simulink model "final"  (R2014a)
settings: Solver=FixedStepDiscrete  StartTime=0.0  StopTime=50000  FixedStep=1  RelTol=1e-3
libraries: hdlsllib x15, simulink x5
settings Model: Creator=you.r  LastModifiedBy=sheehan.pat
settings OptimizationCC: BlockReduction=off  ConditionallyExecuteInputs=off  InlineParams=on
settings DebuggingCC: AlgebraicLoopMsg=error
settings HardwareCC: ProdHWDeviceType=ASIC/FPGA->ASIC/FPGA  ProdEqTarget=off

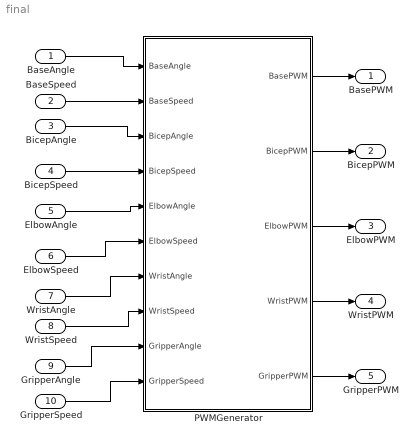
== system final ==
  BaseAngle : Inport
  BaseSpeed : Inport  Port=2
  BicepAngle : Inport  Port=3
  BicepSpeed : Inport  Port=4
  ElbowAngle : Inport  Port=5
  ElbowSpeed : Inport  Port=6
  WristAngle : Inport  Port=7
  WristSpeed : Inport  Port=8
  GripperAngle : Inport  Port=9
  GripperSpeed : Inport  Port=10
  PWMGenerator : Subsystem  TreatAsAtomicUnit=on  SystemSampleTime=1
  BasePWM : Outport  OutDataTypeStr=boolean  SampleTime=1
  BicepPWM : Outport  Port=2  OutDataTypeStr=boolean  SampleTime=1
  ElbowPWM : Outport  Port=3  OutDataTypeStr=boolean  SampleTime=1
  WristPWM : Outport  Port=4  OutDataTypeStr=boolean  SampleTime=1
  GripperPWM : Outport  Port=5  OutDataTypeStr=boolean  SampleTime=1
  wires:
  PWMGenerator/1(BasePWM) -> BasePWM/1
  PWMGenerator/2(BicepPWM) -> BicepPWM/1
  PWMGenerator/3(ElbowPWM) -> ElbowPWM/1
  PWMGenerator/4(WristPWM) -> WristPWM/1
  PWMGenerator/5(GripperPWM) -> GripperPWM/1
  ElbowAngle/1 -> PWMGenerator/5(ElbowAngle)
  ElbowSpeed/1 -> PWMGenerator/6(ElbowSpeed)
  BicepSpeed/1 -> PWMGenerator/4(BicepSpeed)
  BicepAngle/1 -> PWMGenerator/3(BicepAngle)
  WristAngle/1 -> PWMGenerator/7(WristAngle)
  WristSpeed/1 -> PWMGenerator/8(WristSpeed)
  BaseSpeed/1 -> PWMGenerator/2(BaseSpeed)
  BaseAngle/1 -> PWMGenerator/1(BaseAngle)
  GripperAngle/1 -> PWMGenerator/9(GripperAngle)
  GripperSpeed/1 -> PWMGenerator/10(GripperSpeed)

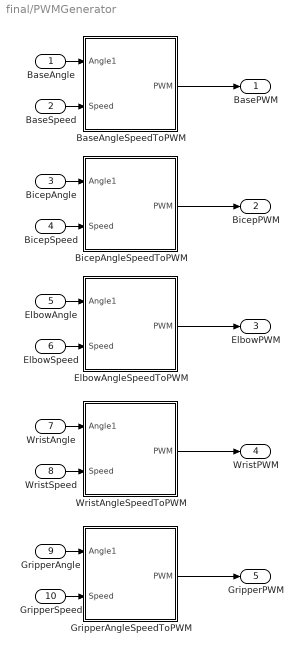
== system final/PWMGenerator ==
  BaseAngle : Inport
  BaseSpeed : Inport  Port=2
  BicepAngle : Inport  Port=3
  BicepSpeed : Inport  Port=4
  ElbowAngle : Inport  Port=5
  ElbowSpeed : Inport  Port=6
  WristAngle : Inport  Port=7
  WristSpeed : Inport  Port=8
  GripperAngle : Inport  Port=9
  GripperSpeed : Inport  Port=10
  BaseAngleSpeedToPWM : Subsystem  TreatAsAtomicUnit=on  SystemSampleTime=1
  BicepAngleSpeedToPWM : Subsystem  TreatAsAtomicUnit=on  SystemSampleTime=1
  ElbowAngleSpeedToPWM : Subsystem  TreatAsAtomicUnit=on  SystemSampleTime=1
  GripperAngleSpeedToPWM : Subsystem  TreatAsAtomicUnit=on  SystemSampleTime=1
  WristAngleSpeedToPWM : Subsystem  TreatAsAtomicUnit=on  SystemSampleTime=1
  BasePWM : Outport  OutDataTypeStr=boolean  SampleTime=1
  BicepPWM : Outport  Port=2  OutDataTypeStr=boolean  SampleTime=1
  ElbowPWM : Outport  Port=3  OutDataTypeStr=boolean  SampleTime=1
  WristPWM : Outport  Port=4  OutDataTypeStr=boolean  SampleTime=1
  GripperPWM : Outport  Port=5  OutDataTypeStr=boolean  SampleTime=1
  wires:
  BaseAngleSpeedToPWM/1(PWM) -> BasePWM/1
  GripperAngleSpeedToPWM/1(PWM) -> GripperPWM/1
  ElbowSpeed/1 -> ElbowAngleSpeedToPWM/2(Speed)
  BaseSpeed/1 -> BaseAngleSpeedToPWM/2(Speed)
  GripperAngle/1 -> GripperAngleSpeedToPWM/1(Angle1)
  WristSpeed/1 -> WristAngleSpeedToPWM/2(Speed)
  BicepSpeed/1 -> BicepAngleSpeedToPWM/2(Speed)
  ElbowAngle/1 -> ElbowAngleSpeedToPWM/1(Angle1)
  GripperSpeed/1 -> GripperAngleSpeedToPWM/2(Speed)
  BaseAngle/1 -> BaseAngleSpeedToPWM/1(Angle1)
  WristAngle/1 -> WristAngleSpeedToPWM/1(Angle1)
  BicepAngle/1 -> BicepAngleSpeedToPWM/1(Angle1)
  BicepAngleSpeedToPWM/1(PWM) -> BicepPWM/1
  ElbowAngleSpeedToPWM/1(PWM) -> ElbowPWM/1
  WristAngleSpeedToPWM/1(PWM) -> WristPWM/1

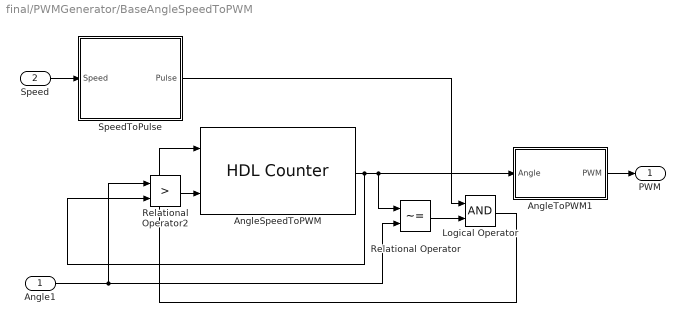
== system final/PWMGenerator/BaseAngleSpeedToPWM ==
  Angle1 : Inport  OutDataTypeStr=uint8
  Speed : Inport  Port=2  OutDataTypeStr=uint8
  AngleSpeedToPWM : hdlsllib/HDL Operations/HDL Counter  CountType=Count limited  CountInit=90  CountStep=1  CountMax=180  CountFromType=Initial value  CountFrom=90  CountResetPort=off  CountLoadPort=off  CountEnbPort=on  CountDirPort=on  CountDataType=Unsigned  CountWordLen=8  CountFracLen=0  CountSampTime=1
  AngleToPWM1 : Subsystem
  Logical Operator : Logic  AllPortsSameDT=off  OutDataTypeStr=boolean
  Relational Operator : RelationalOperator  Operator=~=  OutDataTypeStr=boolean
  Relational Operator2 : RelationalOperator  Operator=>  OutDataTypeStr=boolean
  SpeedToPulse : Subsystem
  PWM : Outport  OutDataTypeStr=boolean  SampleTime=1
  wires:
  Relational Operator/1 -> Logical Operator/2
  AngleSpeedToPWM/1 -> Relational Operator2/2, AngleToPWM1/1(Angle), Relational Operator/1
  Angle1/1 -> Relational Operator2/1, Relational Operator/2
  Relational Operator2/1 -> AngleSpeedToPWM/2
  Logical Operator/1 -> AngleSpeedToPWM/1
  SpeedToPulse/1(Pulse) -> Logical Operator/1
  Speed/1 -> SpeedToPulse/1(Speed)
  AngleToPWM1/1(PWM) -> PWM/1

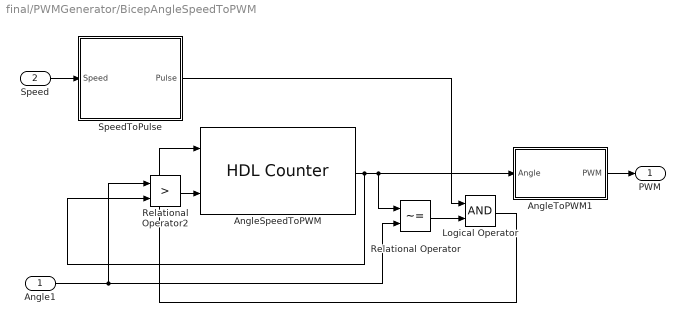
== system final/PWMGenerator/BicepAngleSpeedToPWM ==
  Angle1 : Inport  OutDataTypeStr=uint8
  Speed : Inport  Port=2  OutDataTypeStr=uint8
  AngleSpeedToPWM : hdlsllib/HDL Operations/HDL Counter  CountType=Count limited  CountInit=90  CountStep=1  CountMax=180  CountFromType=Initial value  CountFrom=90  CountResetPort=off  CountLoadPort=off  CountEnbPort=on  CountDirPort=on  CountDataType=Unsigned  CountWordLen=8  CountFracLen=0  CountSampTime=1
  AngleToPWM1 : Subsystem
  Logical Operator : Logic  AllPortsSameDT=off  OutDataTypeStr=boolean
  Relational Operator : RelationalOperator  Operator=~=  OutDataTypeStr=boolean
  Relational Operator2 : RelationalOperator  Operator=>  OutDataTypeStr=boolean
  SpeedToPulse : Subsystem
  PWM : Outport  OutDataTypeStr=boolean  SampleTime=1
  wires:
  Relational Operator/1 -> Logical Operator/2
  AngleSpeedToPWM/1 -> Relational Operator2/2, AngleToPWM1/1(Angle), Relational Operator/1
  Angle1/1 -> Relational Operator2/1, Relational Operator/2
  Relational Operator2/1 -> AngleSpeedToPWM/2
  Logical Operator/1 -> AngleSpeedToPWM/1
  SpeedToPulse/1(Pulse) -> Logical Operator/1
  Speed/1 -> SpeedToPulse/1(Speed)
  AngleToPWM1/1(PWM) -> PWM/1

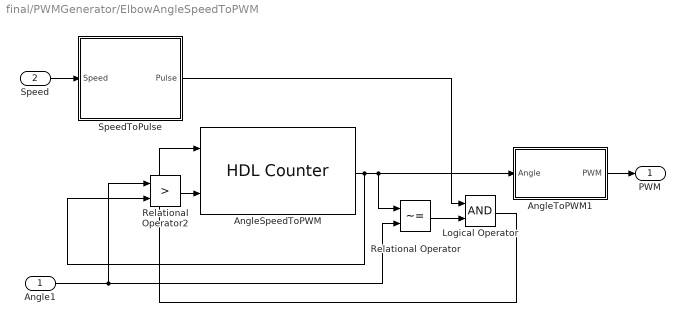
== system final/PWMGenerator/ElbowAngleSpeedToPWM ==
  Angle1 : Inport  OutDataTypeStr=uint8
  Speed : Inport  Port=2  OutDataTypeStr=uint8
  AngleSpeedToPWM : hdlsllib/HDL Operations/HDL Counter  CountType=Count limited  CountInit=90  CountStep=1  CountMax=180  CountFromType=Initial value  CountFrom=90  CountResetPort=off  CountLoadPort=off  CountEnbPort=on  CountDirPort=on  CountDataType=Unsigned  CountWordLen=8  CountFracLen=0  CountSampTime=1
  AngleToPWM1 : Subsystem
  Logical Operator : Logic  AllPortsSameDT=off  OutDataTypeStr=boolean
  Relational Operator : RelationalOperator  Operator=~=  OutDataTypeStr=boolean
  Relational Operator2 : RelationalOperator  Operator=>  OutDataTypeStr=boolean
  SpeedToPulse : Subsystem
  PWM : Outport  OutDataTypeStr=boolean  SampleTime=1
  wires:
  Relational Operator/1 -> Logical Operator/2
  AngleSpeedToPWM/1 -> Relational Operator2/2, AngleToPWM1/1(Angle), Relational Operator/1
  Angle1/1 -> Relational Operator2/1, Relational Operator/2
  Relational Operator2/1 -> AngleSpeedToPWM/2
  Logical Operator/1 -> AngleSpeedToPWM/1
  SpeedToPulse/1(Pulse) -> Logical Operator/1
  Speed/1 -> SpeedToPulse/1(Speed)
  AngleToPWM1/1(PWM) -> PWM/1

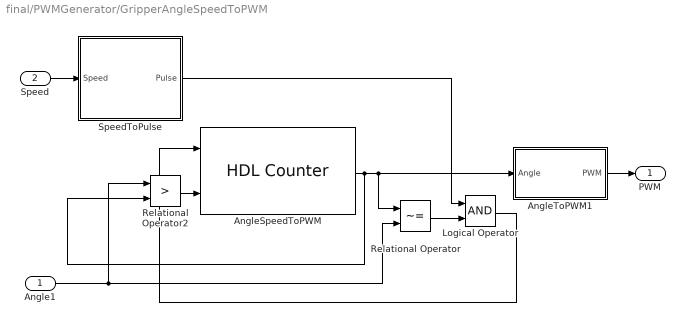
== system final/PWMGenerator/GripperAngleSpeedToPWM ==
  Angle1 : Inport  OutDataTypeStr=uint8
  Speed : Inport  Port=2  OutDataTypeStr=uint8
  AngleSpeedToPWM : hdlsllib/HDL Operations/HDL Counter  CountType=Count limited  CountInit=90  CountStep=1  CountMax=180  CountFromType=Initial value  CountFrom=90  CountResetPort=off  CountLoadPort=off  CountEnbPort=on  CountDirPort=on  CountDataType=Unsigned  CountWordLen=8  CountFracLen=0  CountSampTime=1
  AngleToPWM1 : Subsystem
  Logical Operator : Logic  AllPortsSameDT=off  OutDataTypeStr=boolean
  Relational Operator : RelationalOperator  Operator=~=  OutDataTypeStr=boolean
  Relational Operator2 : RelationalOperator  Operator=>  OutDataTypeStr=boolean
  SpeedToPulse : Subsystem
  PWM : Outport  OutDataTypeStr=boolean  SampleTime=1
  wires:
  Relational Operator/1 -> Logical Operator/2
  AngleSpeedToPWM/1 -> Relational Operator2/2, AngleToPWM1/1(Angle), Relational Operator/1
  Angle1/1 -> Relational Operator2/1, Relational Operator/2
  Relational Operator2/1 -> AngleSpeedToPWM/2
  Logical Operator/1 -> AngleSpeedToPWM/1
  SpeedToPulse/1(Pulse) -> Logical Operator/1
  Speed/1 -> SpeedToPulse/1(Speed)
  AngleToPWM1/1(PWM) -> PWM/1

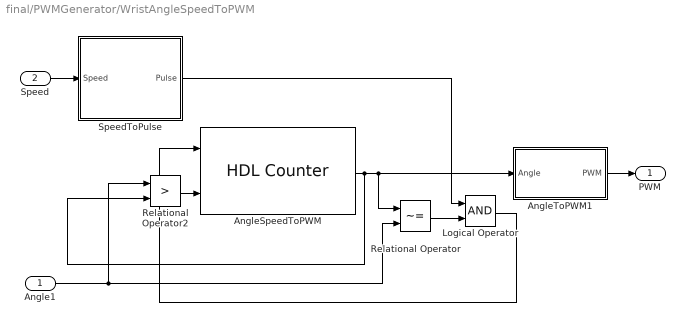
== system final/PWMGenerator/WristAngleSpeedToPWM ==
  Angle1 : Inport  OutDataTypeStr=uint8
  Speed : Inport  Port=2  OutDataTypeStr=uint8
  AngleSpeedToPWM : hdlsllib/HDL Operations/HDL Counter  CountType=Count limited  CountInit=90  CountStep=1  CountMax=180  CountFromType=Initial value  CountFrom=90  CountResetPort=off  CountLoadPort=off  CountEnbPort=on  CountDirPort=on  CountDataType=Unsigned  CountWordLen=8  CountFracLen=0  CountSampTime=1
  AngleToPWM1 : Subsystem
  Logical Operator : Logic  AllPortsSameDT=off  OutDataTypeStr=boolean
  Relational Operator : RelationalOperator  Operator=~=  OutDataTypeStr=boolean
  Relational Operator2 : RelationalOperator  Operator=>  OutDataTypeStr=boolean
  SpeedToPulse : Subsystem
  PWM : Outport  OutDataTypeStr=boolean  SampleTime=1
  wires:
  Relational Operator/1 -> Logical Operator/2
  AngleSpeedToPWM/1 -> Relational Operator2/2, AngleToPWM1/1(Angle), Relational Operator/1
  Angle1/1 -> Relational Operator2/1, Relational Operator/2
  Relational Operator2/1 -> AngleSpeedToPWM/2
  Logical Operator/1 -> AngleSpeedToPWM/1
  SpeedToPulse/1(Pulse) -> Logical Operator/1
  Speed/1 -> SpeedToPulse/1(Speed)
  AngleToPWM1/1(PWM) -> PWM/1

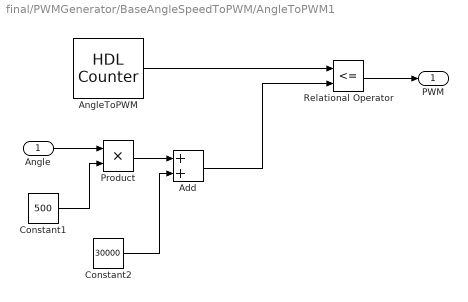
== system final/PWMGenerator/BaseAngleSpeedToPWM/AngleToPWM1 ==
  Angle : Inport  OutDataTypeStr=uint8
  Add : Sum
  AngleToPWM : hdlsllib/HDL Operations/HDL Counter  CountType=Count limited  CountInit=0  CountStep=1  CountMax=1000000  CountFromType=Initial value  CountFrom=0  CountResetPort=off  CountLoadPort=off  CountEnbPort=off  CountDirPort=off  CountDataType=Unsigned  CountWordLen=32  CountFracLen=0  CountSampTime=1
  Constant1 : Constant  Value=500  OutDataTypeStr=uint32  SampleTime=-1
  Constant2 : Constant  Value=30000  OutDataTypeStr=uint32  SampleTime=-1
  Product : Product
  Relational Operator : RelationalOperator  Operator=<=  OutDataTypeStr=boolean
  PWM : Outport
  wires:
  AngleToPWM/1 -> Relational Operator/1
  Angle/1 -> Product/1
  Relational Operator/1 -> PWM/1
  Constant1/1 -> Product/2
  Add/1 -> Relational Operator/2
  Constant2/1 -> Add/2
  Product/1 -> Add/1

== system final/PWMGenerator/BaseAngleSpeedToPWM/SpeedToPulse ==
  Speed : Inport
  Compare To Constant : simulink/Logic and Bit Operations/Compare To Constant  relop===  const=0  OutDataTypeStr=boolean
  Constant : Constant  Value=50000000  OutDataTypeStr=uint32  SampleTime=1
  Divide : Product  Inputs=*/  SaturateOnIntegerOverflow=on  RndMeth=Zero
  HDL Counter : hdlsllib/HDL Operations/HDL Counter  CountType=Free running  CountInit=0  CountStep=1  CountMax=100  CountFromType=Initial value  CountFrom=0  CountResetPort=on  CountLoadPort=off  CountEnbPort=off  CountDirPort=off  CountDataType=Unsigned  CountWordLen=32  CountFracLen=0  CountSampTime=1
  Relational Operator : RelationalOperator  Operator=>  OutDataTypeStr=boolean  SampleTime=1
  Pulse : Outport  OutDataTypeStr=boolean  SampleTime=1
  wires:
  Relational Operator/1 -> HDL Counter/1
  Compare To Constant/1 -> Pulse/1
  Constant/1 -> Divide/1
  Divide/1 -> Relational Operator/2
  HDL Counter/1 -> Relational Operator/1, Compare To Constant/1
  Speed/1 -> Divide/2

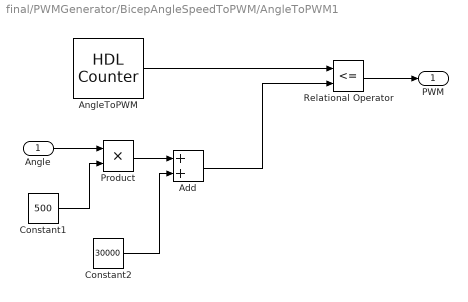
== system final/PWMGenerator/BicepAngleSpeedToPWM/AngleToPWM1 ==
  Angle : Inport  OutDataTypeStr=uint8
  Add : Sum
  AngleToPWM : hdlsllib/HDL Operations/HDL Counter  CountType=Count limited  CountInit=0  CountStep=1  CountMax=1000000  CountFromType=Initial value  CountFrom=0  CountResetPort=off  CountLoadPort=off  CountEnbPort=off  CountDirPort=off  CountDataType=Unsigned  CountWordLen=32  CountFracLen=0  CountSampTime=1
  Constant1 : Constant  Value=500  OutDataTypeStr=uint32  SampleTime=-1
  Constant2 : Constant  Value=30000  OutDataTypeStr=uint32  SampleTime=-1
  Product : Product
  Relational Operator : RelationalOperator  Operator=<=  OutDataTypeStr=boolean
  PWM : Outport
  wires:
  AngleToPWM/1 -> Relational Operator/1
  Angle/1 -> Product/1
  Relational Operator/1 -> PWM/1
  Constant1/1 -> Product/2
  Add/1 -> Relational Operator/2
  Constant2/1 -> Add/2
  Product/1 -> Add/1

== system final/PWMGenerator/BicepAngleSpeedToPWM/SpeedToPulse ==
  Speed : Inport
  Compare To Constant : simulink/Logic and Bit Operations/Compare To Constant  relop===  const=0  OutDataTypeStr=boolean
  Constant : Constant  Value=50000000  OutDataTypeStr=uint32  SampleTime=1
  Divide : Product  Inputs=*/  SaturateOnIntegerOverflow=on  RndMeth=Zero
  HDL Counter : hdlsllib/HDL Operations/HDL Counter  CountType=Free running  CountInit=0  CountStep=1  CountMax=100  CountFromType=Initial value  CountFrom=0  CountResetPort=on  CountLoadPort=off  CountEnbPort=off  CountDirPort=off  CountDataType=Unsigned  CountWordLen=32  CountFracLen=0  CountSampTime=1
  Relational Operator : RelationalOperator  Operator=>  OutDataTypeStr=boolean  SampleTime=1
  Pulse : Outport  OutDataTypeStr=boolean  SampleTime=1
  wires:
  Relational Operator/1 -> HDL Counter/1
  Compare To Constant/1 -> Pulse/1
  Constant/1 -> Divide/1
  Divide/1 -> Relational Operator/2
  HDL Counter/1 -> Relational Operator/1, Compare To Constant/1
  Speed/1 -> Divide/2

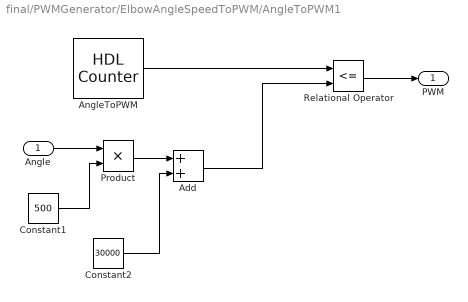
== system final/PWMGenerator/ElbowAngleSpeedToPWM/AngleToPWM1 ==
  Angle : Inport  OutDataTypeStr=uint8
  Add : Sum
  AngleToPWM : hdlsllib/HDL Operations/HDL Counter  CountType=Count limited  CountInit=0  CountStep=1  CountMax=1000000  CountFromType=Initial value  CountFrom=0  CountResetPort=off  CountLoadPort=off  CountEnbPort=off  CountDirPort=off  CountDataType=Unsigned  CountWordLen=32  CountFracLen=0  CountSampTime=1
  Constant1 : Constant  Value=500  OutDataTypeStr=uint32  SampleTime=-1
  Constant2 : Constant  Value=30000  OutDataTypeStr=uint32  SampleTime=-1
  Product : Product
  Relational Operator : RelationalOperator  Operator=<=  OutDataTypeStr=boolean
  PWM : Outport
  wires:
  AngleToPWM/1 -> Relational Operator/1
  Angle/1 -> Product/1
  Relational Operator/1 -> PWM/1
  Constant1/1 -> Product/2
  Add/1 -> Relational Operator/2
  Constant2/1 -> Add/2
  Product/1 -> Add/1

== system final/PWMGenerator/ElbowAngleSpeedToPWM/SpeedToPulse ==
  Speed : Inport
  Compare To Constant : simulink/Logic and Bit Operations/Compare To Constant  relop===  const=0  OutDataTypeStr=boolean
  Constant : Constant  Value=50000000  OutDataTypeStr=uint32  SampleTime=1
  Divide : Product  Inputs=*/  SaturateOnIntegerOverflow=on  RndMeth=Zero
  HDL Counter : hdlsllib/HDL Operations/HDL Counter  CountType=Free running  CountInit=0  CountStep=1  CountMax=100  CountFromType=Initial value  CountFrom=0  CountResetPort=on  CountLoadPort=off  CountEnbPort=off  CountDirPort=off  CountDataType=Unsigned  CountWordLen=32  CountFracLen=0  CountSampTime=1
  Relational Operator : RelationalOperator  Operator=>  OutDataTypeStr=boolean  SampleTime=1
  Pulse : Outport  OutDataTypeStr=boolean  SampleTime=1
  wires:
  Relational Operator/1 -> HDL Counter/1
  Compare To Constant/1 -> Pulse/1
  Constant/1 -> Divide/1
  Divide/1 -> Relational Operator/2
  HDL Counter/1 -> Relational Operator/1, Compare To Constant/1
  Speed/1 -> Divide/2

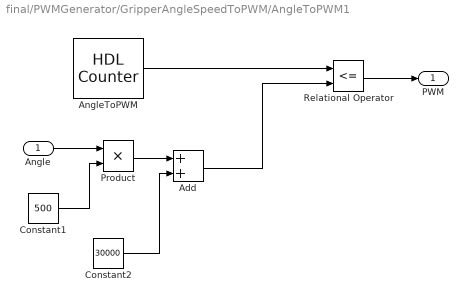
== system final/PWMGenerator/GripperAngleSpeedToPWM/AngleToPWM1 ==
  Angle : Inport  OutDataTypeStr=uint8
  Add : Sum
  AngleToPWM : hdlsllib/HDL Operations/HDL Counter  CountType=Count limited  CountInit=0  CountStep=1  CountMax=1000000  CountFromType=Initial value  CountFrom=0  CountResetPort=off  CountLoadPort=off  CountEnbPort=off  CountDirPort=off  CountDataType=Unsigned  CountWordLen=32  CountFracLen=0  CountSampTime=1
  Constant1 : Constant  Value=500  OutDataTypeStr=uint32  SampleTime=-1
  Constant2 : Constant  Value=30000  OutDataTypeStr=uint32  SampleTime=-1
  Product : Product
  Relational Operator : RelationalOperator  Operator=<=  OutDataTypeStr=boolean
  PWM : Outport
  wires:
  AngleToPWM/1 -> Relational Operator/1
  Angle/1 -> Product/1
  Relational Operator/1 -> PWM/1
  Constant1/1 -> Product/2
  Add/1 -> Relational Operator/2
  Constant2/1 -> Add/2
  Product/1 -> Add/1

== system final/PWMGenerator/GripperAngleSpeedToPWM/SpeedToPulse ==
  Speed : Inport
  Compare To Constant : simulink/Logic and Bit Operations/Compare To Constant  relop===  const=0  OutDataTypeStr=boolean
  Constant : Constant  Value=50000000  OutDataTypeStr=uint32  SampleTime=1
  Divide : Product  Inputs=*/  SaturateOnIntegerOverflow=on  RndMeth=Zero
  HDL Counter : hdlsllib/HDL Operations/HDL Counter  CountType=Free running  CountInit=0  CountStep=1  CountMax=100  CountFromType=Initial value  CountFrom=0  CountResetPort=on  CountLoadPort=off  CountEnbPort=off  CountDirPort=off  CountDataType=Unsigned  CountWordLen=32  CountFracLen=0  CountSampTime=1
  Relational Operator : RelationalOperator  Operator=>  OutDataTypeStr=boolean  SampleTime=1
  Pulse : Outport  OutDataTypeStr=boolean  SampleTime=1
  wires:
  Relational Operator/1 -> HDL Counter/1
  Compare To Constant/1 -> Pulse/1
  Constant/1 -> Divide/1
  Divide/1 -> Relational Operator/2
  HDL Counter/1 -> Relational Operator/1, Compare To Constant/1
  Speed/1 -> Divide/2

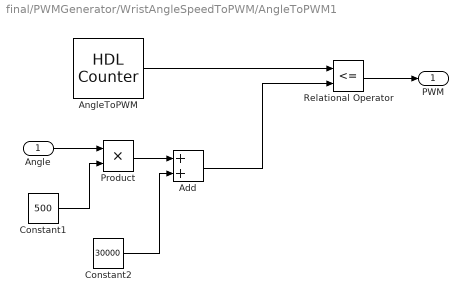
== system final/PWMGenerator/WristAngleSpeedToPWM/AngleToPWM1 ==
  Angle : Inport  OutDataTypeStr=uint8
  Add : Sum
  AngleToPWM : hdlsllib/HDL Operations/HDL Counter  CountType=Count limited  CountInit=0  CountStep=1  CountMax=1000000  CountFromType=Initial value  CountFrom=0  CountResetPort=off  CountLoadPort=off  CountEnbPort=off  CountDirPort=off  CountDataType=Unsigned  CountWordLen=32  CountFracLen=0  CountSampTime=1
  Constant1 : Constant  Value=500  OutDataTypeStr=uint32  SampleTime=-1
  Constant2 : Constant  Value=30000  OutDataTypeStr=uint32  SampleTime=-1
  Product : Product
  Relational Operator : RelationalOperator  Operator=<=  OutDataTypeStr=boolean
  PWM : Outport
  wires:
  AngleToPWM/1 -> Relational Operator/1
  Angle/1 -> Product/1
  Relational Operator/1 -> PWM/1
  Constant1/1 -> Product/2
  Add/1 -> Relational Operator/2
  Constant2/1 -> Add/2
  Product/1 -> Add/1

== system final/PWMGenerator/WristAngleSpeedToPWM/SpeedToPulse ==
  Speed : Inport
  Compare To Constant : simulink/Logic and Bit Operations/Compare To Constant  relop===  const=0  OutDataTypeStr=boolean
  Constant : Constant  Value=50000000  OutDataTypeStr=uint32  SampleTime=1
  Divide : Product  Inputs=*/  SaturateOnIntegerOverflow=on  RndMeth=Zero
  HDL Counter : hdlsllib/HDL Operations/HDL Counter  CountType=Free running  CountInit=0  CountStep=1  CountMax=100  CountFromType=Initial value  CountFrom=0  CountResetPort=on  CountLoadPort=off  CountEnbPort=off  CountDirPort=off  CountDataType=Unsigned  CountWordLen=32  CountFracLen=0  CountSampTime=1
  Relational Operator : RelationalOperator  Operator=>  OutDataTypeStr=boolean  SampleTime=1
  Pulse : Outport  OutDataTypeStr=boolean  SampleTime=1
  wires:
  Relational Operator/1 -> HDL Counter/1
  Compare To Constant/1 -> Pulse/1
  Constant/1 -> Divide/1
  Divide/1 -> Relational Operator/2
  HDL Counter/1 -> Relational Operator/1, Compare To Constant/1
  Speed/1 -> Divide/2
